simulink model "quarc_py_bridge_bb"  (Simulink 8.9)
settings: Solver=ode1  StartTime=0.0  StopTime=inf  FixedStep=0.002  RelTol=1e-3  EnableMultiTasking=on
InitFcn:
  | load bus_object_bb.mat
undefined symbols (not defined in the file or in its folder): HIL, qc_get_step_size
libraries: quarc_library x9, simulink x1
settings Model: Creator=MLevis  LastModifiedBy=Quanser  SimulationMode=external  ExtModeTrigDuration=5000
settings SolverCC: PositivePriorityOrder=on
settings OptimizationCC: ExpressionDepthLimit=2147483647
settings DebuggingCC: SolverPrmCheckMsg=warning
settings RTWCC: SystemTargetFile=quarc_win64.tlc  TemplateMakefile=quarc_default_tmf  Description=QUARC Win64 Target
settings STFCustomTargetCC: TargetPreCompLibLocation=C:\PROGRA~3\QUARC\lib\2017a\win64\release  ConcurrentExecutionCompliant=on  GeneratePreprocessorConditionals=Disable all  SystemTargetFile=quarc_win64.tlc
settings GRTTargetCC: TargetPreCompLibLocation=C:\PROGRA~3\QUARC\lib\2017a\win64\release  ParMdlRefBuildCompliant=off  CompOptLevelCompliant=off  MatFileLogging=off  CPPClassGenCompliant=off  UseToolchainInfoCompliant=off  ExtMode=on  ExtModeMexFile=quarc_comm
settings ConfigComp: CovSFcnEnable=off

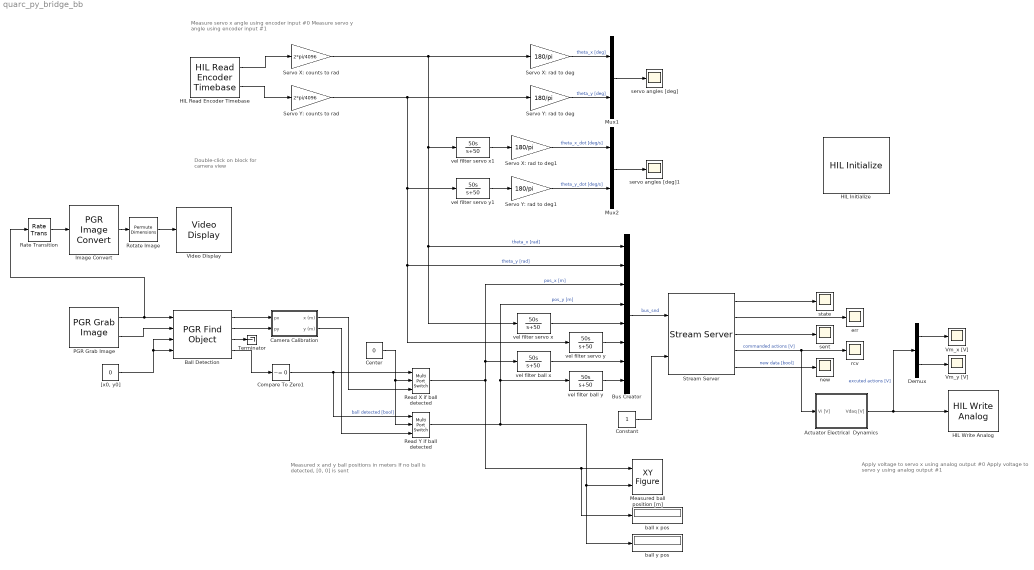
== system quarc_py_bridge_bb ==
  note: Measured x and y ball positions in meters
      | If no ball is detected, [0, 0] is sent
  note: Measure servo x angle using encoder input #0
      | Measure servo y angle using encoder input #1
  note: Apply voltage to servo x using analog output #0
      | Apply voltage to servo y using analog output #1
  note: Double-click on block
      | for camera view
  " Rotate Image" : PermuteDimensions  Order=[2,1,3]
  Actuator Electrical  Dynamics : Subsystem
  Ball Detection : quarc_library/Image Processing/Point Grey Research/PGR Find Object  detect_mode=RGB  pixel_format=BGR8  num_objects=1  lum_threshold=50  min_size=500  r_value=250  g_value=125  b_value=50  sample_time=-1
      settings: SourceProductName=QUARC Targets
  Bus Creator : BusCreator  Inputs=8
  Camera Calibration : Subsystem
  Center : Constant  Value=0
  Compare To Zero1 : simulink/Logic and Bit Operations/Compare To Zero  relop=~=  OutDataTypeStr=boolean
  Constant : Constant
  Demux : Demux  Outputs=2
  HIL Initialize : quarc_library/Data Acquisition/Generic/Configuration/HIL Initialize  object_name=HIL-1  board_type=q8_usb  board_number=0  board_options=update_rate=normal;decimation=1  exclusive=off  active=on  hardware_clocks=[0:2]  clock_modes=[]  initial_clock_frequencies=[]  set_clock_params_at_start=off  set_clock_params_at_switch_in=off  set_clock_frequencies_at_start=off  set_clock_frequencies_at_switch_in=off  analog_input_channels=[0:7]  analog_input_configurations=[]  analog_input_maximums=10  analog_input_minimums=-10  set_analog_input_params_at_start=on  set_analog_input_params_at_switch_in=off  analog_output_channels=[0:7]  analog_output_maximums=10  analog_output_minimums=-10  initial_analog_outputs=[0]  final_analog_outputs=[0]  watchdog_analog_outputs=0  set_analog_output_params_at_start=on  set_analog_output_params_at_switch_in=off  set_analog_outputs_at_start=on  set_analog_outputs_at_switch_in=off  set_analog_outputs_at_terminate=on  set_analog_outputs_at_switch_out=off  set_analog_outputs_on_watchdog=off  digital_input_channels=[]  digital_output_channels=[0:7]  digital_output_configuration=[]  initial_digital_outputs=[1]  final_digital_outputs=[0]  watchdog_digital_outputs=[0]  set_digital_output_params_at_start=off  set_digital_output_params_at_switch_in=off  set_digital_outputs_at_start=on  set_digital_outputs_at_switch_in=off  set_digital_outputs_at_terminate=on  set_digital_outputs_at_switch_out=off  set_digital_outputs_on_watchdog=off  encoder_channels=[0:7]  quadrature=[4]  encoder_filter_frequency=[]  initial_encoder_counts=[0]  set_encoder_params_at_start=on  set_encoder_params_at_switch_in=off  set_encoder_counts_at_start=on  set_encoder_counts_at_switch_in=off  pwm_channels=[0:7]  pwm_modes=0  pwm_frequency=99.532799999999995e6/4095  pwm_configuration=[0]  pwm_alignment=[0]  pwm_polarity=[1]  pwm_leading_deadband=[0]  pwm_trailing_deadband=[0]  initial_pwm_outputs=[0]  final_pwm_outputs=[0]  watchdog_pwm_outputs=[0]  set_pwm_params_at_start=on  set_pwm_params_at_switch_in=off  set_pwm_outputs_at_start=on  set_pwm_outputs_at_switch_in=off  set_pwm_outputs_at_terminate=on  set_pwm_outputs_at_switch_out=off  set_pwm_outputs_on_watchdog=off  other_output_channels=[]  initial_other_outputs=[]  final_other_outputs=[]  watchdog_other_outputs=[]  set_other_outputs_at_start=off  set_other_outputs_at_switch_in=off  set_other_outputs_at_terminate=off  set_other_outputs_at_switch_out=off  set_other_outputs_on_watchdog=off
      settings: AttributesFormatString=(%<object_name>)
  HIL Read Encoder Timebase : quarc_library/Data Acquisition/Generic/Timebases/HIL Read Encoder Timebase  object_name=HIL-1  clock=0  channels=[0:1]  samples_in_buffer=max(ceil(1/qc_get_step_size), 1)  active=on  vector_output=off  data_type_mode=Inherit via back propagation  data_type=double
  HIL Write Analog : quarc_library/Data Acquisition/Generic/Immediate I//O/HIL Write Analog  Tag=unassigned  object_name=HIL-1  channels=[0:1]  sample_time=-1  active=off  vector_input=on
  Image Convert : quarc_library/Image Processing/Point Grey Research/PGR Image Convert  pixel_format=BGR8  convert_mode=Matlab RGB  sample_time=0.1
      settings: SourceProductName=QUARC Targets
  Measured ball position [m] : quarc_library/Sinks/Figures/XY Figure  figure_mode=Use figure window  figure_tag=figure1  axes_tag=axes1  minimum_x=-0.13001  maximum_x=0.13001  minimum_y=-0.13001  maximum_y=0.13001  buffer_size=1000  update_rate=100  initial_position="800  142  958  709"  initial_visibility=off  sample_time=-1
      settings: SourceProductName=QUARC Targets
  Mux1 : Mux  Inputs=2
  Mux2 : Mux  Inputs=2
  PGR Grab Image : quarc_library/Devices/Third-Party/Point Grey Research/Cameras/PGR Grab Image  camera_type=FireflyMV  serial_number=-1  video_mode=Custom Mode  frame_rate=30  left_pos=140  top_pos=20  image_width=440  image_height=440  reset_camera_settings=off  thread_priority=0  sample_time=qc_get_step_size
      settings: SourceProductName=QUARC Targets
  Rate Transition : RateTransition
  Read X if ball detected : MultiPortSwitch  DataPortOrder=Zero-based contiguous  Inputs=2  zeroidx=on
  Read Y if ball detected : MultiPortSwitch  DataPortOrder=Zero-based contiguous  Inputs=2  zeroidx=on
  Servo X: counts to rad : Gain  Gain=2*pi/4096  SaturateOnIntegerOverflow=on  OutDataTypeStr=Inherit: Same as input  ParamDataTypeStr=Inherit: Same as input
  Servo X: rad to deg : Gain  Gain=180/pi  SaturateOnIntegerOverflow=on  OutDataTypeStr=Inherit: Same as input  ParamDataTypeStr=Inherit: Same as input
  Servo X: rad to deg1 : Gain  Gain=180/pi  SaturateOnIntegerOverflow=on  OutDataTypeStr=Inherit: Same as input  ParamDataTypeStr=Inherit: Same as input
  Servo Y: counts to rad : Gain  Gain=2*pi/4096  SaturateOnIntegerOverflow=on  OutDataTypeStr=Inherit: Same as input  ParamDataTypeStr=Inherit: Same as input
  Servo Y: rad to deg : Gain  Gain=180/pi  SaturateOnIntegerOverflow=on  OutDataTypeStr=Inherit: Same as input  ParamDataTypeStr=Inherit: Same as input
  Servo Y: rad to deg1 : Gain  Gain=180/pi  SaturateOnIntegerOverflow=on  OutDataTypeStr=Inherit: Same as input  ParamDataTypeStr=Inherit: Same as input
  Stream Server : quarc_library/Communications/Basic/Stream Server  uri_source=Specify via dialog (do not evaluate)  uri=tcpip://localhost:9095  apply_uri_to_all_configs=on  send_buffer_size=1460  receive_buffer_size=1460  byte_order=big endian (Motorola - MSB first)  optimization=Minimum latency  send_options=Send most recent data  receive_options=Receive most recent data  default_value=[0, 0]  sample_time=qc_get_step_size  active=off  implementation=Use blocking I/O in a separate thread  send_fifo_size=1  receive_fifo_size=1  send_priority=0  receive_priority=0  send_dimensions=off  receive_dimensions=off  max_dimensions=-1  data_type=double  type_expr=BusObject
      settings: AttributesFormatString="\"tcpip://localhost:9095\""
  Terminator : Terminator
  Video Display : quarc_library/Multimedia/Video Display  sample_time=-1  use_hardware=on
  Vm_x [V] : Scope
  Vm_y [V] : Scope
  "[x0, y0]" : Constant  Value=0
  ball x pos : Display
  ball y pos : Display
  err : Scope
  new : Scope
  rcv : Scope
  sent : Scope
  servo angles [deg] : Scope
  servo angles [deg]1 : Scope
  state : Scope
  vel filter ball x : TransferFcn  Numerator=[50 0]  Denominator=[1 50]
  vel filter ball y : TransferFcn  Numerator=[50 0]  Denominator=[1 50]
  vel filter servo x : TransferFcn  Numerator=[50 0]  Denominator=[1 50]
  vel filter servo x1 : TransferFcn  Numerator=[50 0]  Denominator=[1 50]
  vel filter servo y : TransferFcn  Numerator=[50 0]  Denominator=[1 50]
  vel filter servo y1 : TransferFcn  Numerator=[50 0]  Denominator=[1 50]
  wires:
  Stream Server/4 -> Actuator Electrical  Dynamics/1(Vi [V]), rcv/1  "commanded actions [V]"
  Stream Server/5 -> new/1  "new data [bool]"
  Stream Server/3 -> sent/1
  Stream Server/1 -> state/1
  Stream Server/2 -> err/1
  Center/1 -> Read X if ball detected/2, Read Y if ball detected/2
  Camera Calibration/2(y (m)) -> Read Y if ball detected/3
  Compare To Zero1/1 -> Read X if ball detected/1, Read Y if ball detected/1  "ball detected [bool]"
  Bus Creator/1 -> Stream Server/1  "bus_snd"
  HIL Read Encoder Timebase/2 -> Servo Y: counts to rad/1
  Servo X: counts to rad/1 -> vel filter servo x/1, Bus Creator/1, vel filter servo x1/1, Servo X: rad to deg/1  "theta_x [rad]"
  Servo Y: counts to rad/1 -> Servo Y: rad to deg/1, vel filter servo y1/1, Bus Creator/2, vel filter servo y/1  "theta_y [rad]"
  "[x0, y0]"/1 -> Ball Detection/4, Ball Detection/3
  Ball Detection/3 -> Terminator/1
  PGR Grab Image/1 -> Rate Transition/1, Ball Detection/1
  Camera Calibration/1(x (m)) -> Read X if ball detected/3
  Ball Detection/4 -> Compare To Zero1/1
  HIL Read Encoder Timebase/1 -> Servo X: counts to rad/1
  Ball Detection/1 -> Camera Calibration/1(px)
  Ball Detection/2 -> Camera Calibration/2(py)
  Read X if ball detected/1 -> ball x pos/1, Measured ball position [m]/1, Bus Creator/3, vel filter ball x/1  "pos_x [m]"
  PGR Grab Image/2 -> Ball Detection/2
  Actuator Electrical  Dynamics/1(Vdaq [V]) -> HIL Write Analog/1, Demux/1  "excuted actions [V]"
  Demux/1 -> Vm_x [V]/1
  Demux/2 -> Vm_y [V]/1
  Rate Transition/1 -> Image Convert/1
  " Rotate Image"/1 -> Video Display/1
  Image Convert/1 -> " Rotate Image"/1
  Read Y if ball detected/1 -> ball y pos/1, Measured ball position [m]/2, Bus Creator/4, vel filter ball y/1  "pos_y [m]"
  Mux1/1 -> servo angles [deg]/1
  Servo X: rad to deg/1 -> Mux1/1  "theta_x [deg]"
  Servo Y: rad to deg/1 -> Mux1/2  "theta_y [deg]"
  Constant/1 -> Stream Server/2
  vel filter ball x/1 -> Bus Creator/7
  vel filter ball y/1 -> Bus Creator/8
  vel filter servo y/1 -> Bus Creator/6
  vel filter servo x/1 -> Bus Creator/5
  Servo Y: rad to deg1/1 -> Mux2/2  "theta_y_dot [deg/s]"
  Servo X: rad to deg1/1 -> Mux2/1  "theta_x_dot [deg/s]"
  Mux2/1 -> servo angles [deg]1/1
  vel filter servo x1/1 -> Servo X: rad to deg1/1
  vel filter servo y1/1 -> Servo Y: rad to deg1/1

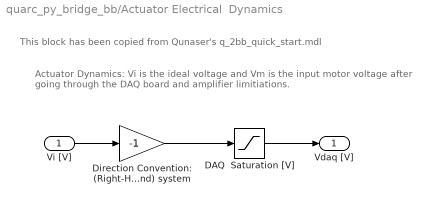
== system quarc_py_bridge_bb/Actuator Electrical  Dynamics ==
  note: Actuator Dynamics: Vi is the ideal voltage and Vm is the
      | input motor voltage after going through the DAQ board and amplifier limitiations.
  note: This block has been copied from Qunaser's q_2bb_quick_start.mdl
  Vi [V] : Inport
  DAQ  Saturation [V] : Saturate  UpperLimit=10  LowerLimit=-10
  Direction Convention: (Right-Hand) system : Gain  Gain=-1  SaturateOnIntegerOverflow=on  OutDataTypeStr=Inherit: Same as input  ParamDataTypeStr=Inherit: Same as input
  Vdaq [V] : Outport
  wires:
  Vi [V]/1 -> Direction Convention: (Right-Hand) system/1
  DAQ  Saturation [V]/1 -> Vdaq [V]/1
  Direction Convention: (Right-Hand) system/1 -> DAQ  Saturation [V]/1

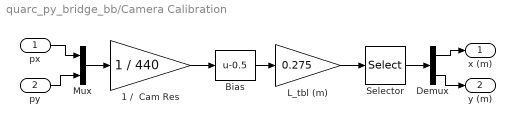
== system quarc_py_bridge_bb/Camera Calibration ==
  px : Inport
  py : Inport  Port=2
  1 /  Cam Res : Gain  Gain=1 / 440
  Bias : Bias  Bias=-0.5
  Demux : Demux  Outputs=2
  L_tbl (m) : Gain  Gain=0.275
  Mux : Mux  Inputs=2
  Selector : Selector  InputPortWidth=2  IndexOptions=Index vector (dialog)  Indices=[2 1]  OutputSizes=1
  x (m) : Outport
  y (m) : Outport  Port=2
  wires:
  Demux/2 -> y (m)/1
  Demux/1 -> x (m)/1
  Selector/1 -> Demux/1
  L_tbl (m)/1 -> Selector/1
  Mux/1 -> 1 /  Cam Res/1
  py/1 -> Mux/2
  px/1 -> Mux/1
  1 /  Cam Res/1 -> Bias/1
  Bias/1 -> L_tbl (m)/1
